simulink model "simTurning_35_Ramp"  (R2020b)
settings: Solver=FixedStepAuto  StartTime=0.0  StopTime=3000.0  FixedStep=0.02  RelTol=1e-3
undefined symbols (not defined in the file or in its folder): p
libraries: simulink x1
settings Model: Creator=teora  LastModifiedBy=teora

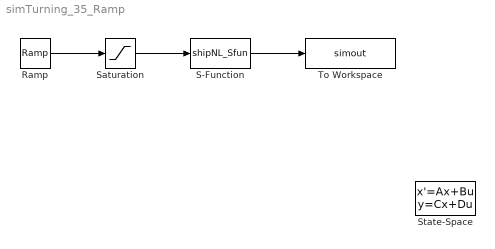
== system simTurning_35_Ramp ==
  Ramp : simulink/Sources/Ramp  slope=p.dDelta  start=0  InitialOutput=0
  S-Function : S-Function  FunctionName=shipNL_Sfun  Parameters=p  SFunctionDeploymentMode=off  EnableBusSupport=off
  Saturation : Saturate  UpperLimit=35*pi/180  LowerLimit=0
  State-Space : StateSpace  InitialCondition=0
  To Workspace : ToWorkspace  VariableName=simout  SaveFormat=Timeseries  SampleTime=-1
  wires:
  S-Function/1 -> To Workspace/1
  Ramp/1 -> Saturation/1
  Saturation/1 -> S-Function/1
